simulink subsystem "StateMachine"  (R2024a)
settings: Solver=VariableStepAuto  StartTime=0.0  StopTime=10.0  RelTol=1e-3
values from neighbouring files (symbols this model uses):
  main_switch = Simulink.Parameter    [LAFES_saveas.m]
  motor_e_stop = Simulink.Parameter    [LAFES_saveas.m]
  quick_stop = Simulink.Parameter    [LAFES_saveas.m]
settings Model: Creator=20192648  LastModifiedBy=20192648
settings ConfigComp: CovBoundaryAbsTol=1.0e-5

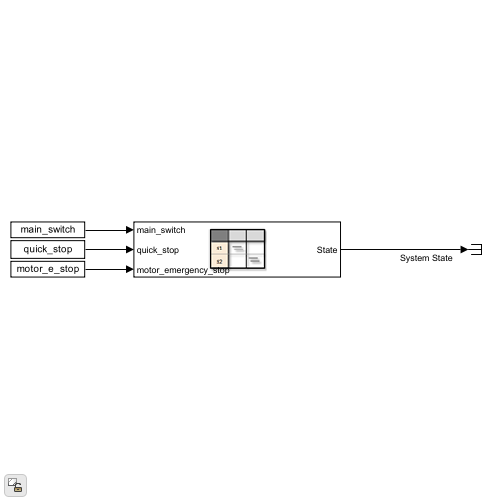
[thumbnail: Simulink's stored preview of the top-level diagram]
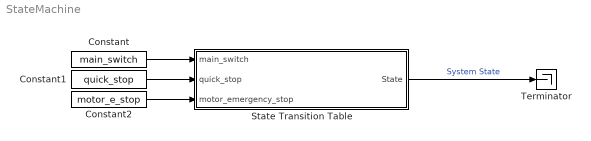
== system StateMachine ==
  Constant : Constant  Value=main_switch
  Constant1 : Constant  Value=quick_stop
  Constant2 : Constant  Value=motor_e_stop
  State Transition Table : State Transition Table  TreatAsAtomicUnit=on
  Terminator : Terminator
  wires:
  Constant/1 -> State Transition Table/1(main_switch)
  State Transition Table/1(State) -> Terminator/1  "System State"
  Constant1/1 -> State Transition Table/2(quick_stop)
  Constant2/1 -> State Transition Table/3(motor_emergency_stop)

== stateflow chart StateMachine/State Transition Table ==
  state Idle
  state Running
  state Quick_Stopping
  state Stopped
  (default) -> Idle
  (junction 52) -> Idle
  (junction 54) -> (junction 52)
  Idle -> Running : [main_switch == true]
  Running -> Idle [order 1] : [main_switch == false]
  Running -> (junction 37) [order 3] : [motor_emergency_stop == true]
  (junction 37) -> (junction 35)
  Running -> Quick_Stopping [order 2] : [quick_stop == true]
  Quick_Stopping -> Running [order 2] : [quick_stop == false]
  Quick_Stopping -> (junction 54) [order 1] : [main_switch == false]
  (junction 35) -> Stopped
  data: main_switch input; State output Enum: State_Transition_TableModeType; quick_stop input; motor_emergency_stop input
